simulink model "Copy_of_simple_model_2017"  (R2017a)
settings: Solver=VariableStepAuto  StartTime=0.0  StopTime=inf  RelTol=1e-3
settings Model: Creator=aboudy  LastModifiedBy=aboudy

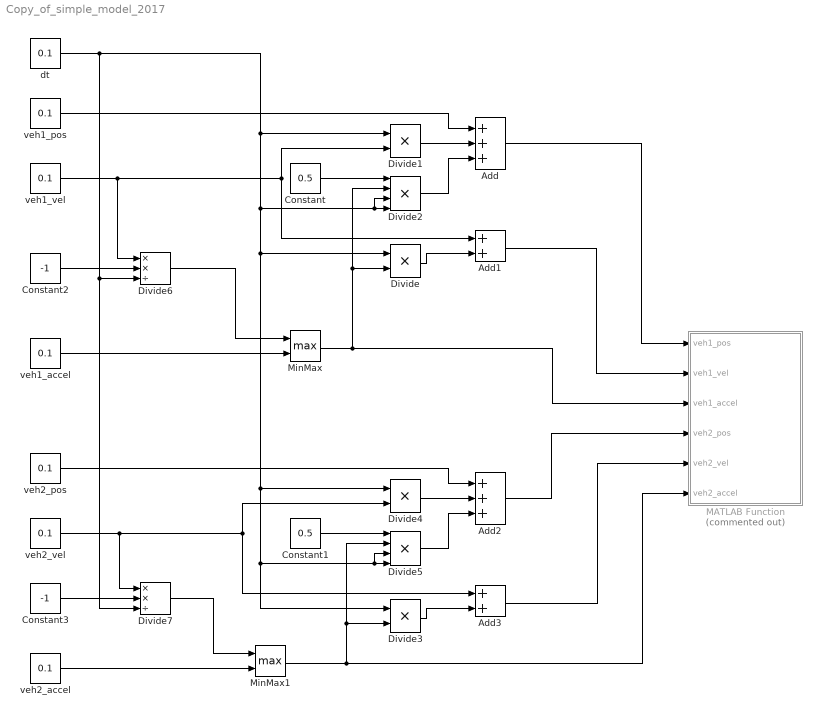
== system Copy_of_simple_model_2017 ==
  Add : Sum  Inputs=+++
  Add1 : Sum
  Add2 : Sum  Inputs=+++
  Add3 : Sum
  Constant : Constant  Value=0.5
  Constant1 : Constant  Value=0.5
  Constant2 : Constant  Value=-1
  Constant3 : Constant  Value=-1
  Divide{,1,3..4} (4 alike) : Product  Inputs=**
  Divide2 : Product  Inputs=****
  Divide5 : Product  Inputs=****
  Divide6 : Product  Inputs=**/
  Divide7 : Product  Inputs=**/
  MATLAB Function : MATLAB Function  Commented=on  TreatAsAtomicUnit=on
  MinMax : MinMax  Function=max  Inputs=2
  MinMax1 : MinMax  Function=max  Inputs=2
  dt : Constant  Value=0.1
  veh1_accel : Constant  Value=0.1
  veh1_pos : Constant  Value=0.1
  veh1_vel : Constant  Value=0.1
  veh2_accel : Constant  Value=0.1
  veh2_pos : Constant  Value=0.1
  veh2_vel : Constant  Value=0.1
  wires:
  Add/1 -> MATLAB Function/1(veh1_pos)
  Add1/1 -> MATLAB Function/2(veh1_vel)
  veh1_vel/1 -> Add1/1, Divide1/2, Divide6/1
  Divide/1 -> Add1/2
  veh1_pos/1 -> Add/1
  Divide1/1 -> Add/2
  Constant/1 -> Divide2/1
  Divide2/1 -> Add/3
  Divide4/1 -> Add2/2
  dt/1 -> Divide7/3, Divide6/3, Divide1/1, Divide/1, Divide4/1, Divide3/1, Divide5/3, Divide5/4, Divide2/3, Divide2/4
  Add3/1 -> MATLAB Function/5(veh2_vel)
  Divide3/1 -> Add3/2
  veh2_accel/1 -> MinMax1/2
  veh2_vel/1 -> Divide4/2, Add3/1, Divide7/1
  Divide5/1 -> Add2/3
  Constant1/1 -> Divide5/1
  Add2/1 -> MATLAB Function/4(veh2_pos)
  veh2_pos/1 -> Add2/1
  MinMax/1 -> Divide2/2, Divide/2, MATLAB Function/3(veh1_accel)
  Constant2/1 -> Divide6/2
  Constant3/1 -> Divide7/2
  MinMax1/1 -> Divide3/2, Divide5/2, MATLAB Function/6(veh2_accel)
  veh1_accel/1 -> MinMax/2
  Divide6/1 -> MinMax/1
  Divide7/1 -> MinMax1/1

== matlab function Copy_of_simple_model_2017/MATLAB Function ==
  data: veh1_pos input; veh1_vel input; veh1_accel input; veh2_pos input; veh2_vel input; veh2_accel input
function fcn(veh1_pos, veh1_vel, veh1_accel, veh2_pos, veh2_vel, veh2_accel)

coder.extrinsic('bdroot')
coder.extrinsic('set_param')
coder.extrinsic('strcat')
coder.extrinsic('strsplit')
coder.extrinsic('string')
coder.extrinsic('num2str')
coder.extrinsic('tcpip')
coder.extrinsic('fopen')
coder.extrinsic('fwrite')
coder.extrinsic('fclose')
coder.extrinsic('fscanf')
coder.extrinsic('mxArrayToString')

coder.extrinsic('class')

% name of model
model = "Copy_of_simple_model_2017";

% steup a tcp/ip connection with python
server = tcpip('localhost', 50005);
fopen(server);

% new state information
veh1_pos = veh1_pos(end);
veh2_pos = veh2_pos(end);
veh1_vel = veh1_vel(end);
veh2_vel = veh2_vel(end);
veh1_accel = veh1_accel(end);
veh2_accel = veh2_accel(end);

% send new state values to Python through the tcp socket
out_data = strcat(num2str(veh1_pos), ":", num2str(veh1_vel), ":", ...
    num2str(veh1_accel), ":", num2str(veh2_pos), ":", ...
    num2str(veh2_vel), ":", num2str(veh2_accel));
fwrite(server, out_data)

% get the next set of actions, and whether the rollout should be
% terminated
in_data = ' -.--: -.--:- ';
in_data = fscanf(server);

% close the tcp/ip connection
fclose(server);

% determine whether the simulation should be termianted
done = (in_data(end-1)=='1');

if done
    set_param(bdroot,'SimulationCommand','stop')
else
    % acceleration of truck 1
    if in_data(1) == ' '
        veh1_accel = in_data(2:5);
    else
        veh1_accel = in_data(1:5);
    end

    % acceleration of truck 2
    if in_data(7) == ' '
        veh2_accel = in_data(8:11);
    else
        veh2_accel = in_data(7:11);
    end

    % update the parameters in the simulink model
    set_param(strcat(model, "/veh1_pos"), "Value", string(veh1_pos))
    set_param(strcat(model, "/veh1_vel"), "Value", string(veh1_vel))
    set_param(strcat(model, "/veh2_pos"), "Value", string(veh2_pos))
    set_param(strcat(model, "/veh2_vel"), "Value", string(veh2_vel))
    set_param(strcat(model, "/veh1_accel"), "Value", string(veh1_accel))
    set_param(strcat(model, "/veh2_accel"), "Value", string(veh2_accel))
end

end
